simulink model "DC_motor_pos"  (R2018b)
settings: Solver=VariableStepAuto  StartTime=0.0  StopTime=10  RelTol=1e-3
settings Model: Creator=EMiR  LastModifiedBy=EMiR
settings SolverCC: ZeroCrossAlgorithm=Adaptive
settings DebuggingCC: IgnoredZcDiagnostic=none

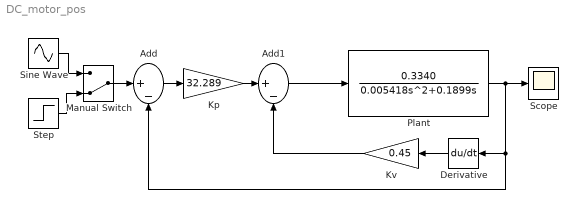
== system DC_motor_pos ==
  Add : Sum  Inputs=|+-
  Add1 : Sum  Inputs=|+-
  Derivative : Derivative
  Kp : Gain  Gain=32.289
  Kv : Gain  Gain=0.45
  Manual Switch : ManualSwitch  CurrentSetting=0
  Plant : TransferFcn  Numerator=[0.3340]  Denominator=[0.005418 0.1899 0]
  Scope : Scope
  Sine Wave : Sin  Amplitude=11  SampleTime=0
  Step : Step  After=11  SampleTime=0  ZeroCross=off
  wires:
  Add/1 -> Kp/1
  Plant/1 -> Scope/1, Add/2, Derivative/1
  Derivative/1 -> Kv/1
  Kv/1 -> Add1/2
  Kp/1 -> Add1/1
  Manual Switch/1 -> Add/1
  Sine Wave/1 -> Manual Switch/1
  Step/1 -> Manual Switch/2
  Add1/1 -> Plant/1
